simulink model "stellaris_test_buttons"  (R2012b)
settings: Solver=FixedStepDiscrete  SolverMode=SingleTasking  StartTime=0.0  StopTime=10.0  FixedStep=0.05  RelTol=1e-3
libraries: stellaris_lib x6, simulink x3
settings Model: Creator=peselnikmg  LastModifiedBy=peselnikmg
settings DataIOCC: SignalLoggingSaveFormat=ModelDataLogs
settings OptimizationCC: OptimizeModelRefInitCode=on  LifeSpan=1
settings HardwareCC: ProdEndianess=LittleEndian  ProdHWDeviceType=Texas Instruments->TMS470
settings RTWCC: SystemTargetFile=stellaris.tlc  TemplateMakefile=stellaris_tmf  PostCodeGenCommand=stellaris_customcode(buildInfo)  Description=TI Stellaris LaunchPad  GenerateReport=on  ProcessScript=stellaris_make_rtw_hook  IncludeHyperlinkInReport=on  GenerateTraceInfo=on  GenerateTraceReport=on  GenerateTraceReportSl=on  GenerateTraceReportSf=on  GenerateTraceReportEml=on  GenerateCodeMetricsReport=on  GenerateCodeReplacementReport=on
settings CodeAppCC: IgnoreCustomStorageClasses=off
settings STFCustomTargetCC: CodeReplacementLibrary=ANSI_C  CombineOutputUpdateFcns=on  ERTCustomFileBanners=on  SupportContinuousTime=off  SupportNonInlinedSFcns=off  GRTInterface=off  SystemTargetFile=stellaris.tlc
settings ERTTargetCC: CodeReplacementLibrary=ANSI_C  MultiwordLength=2048  ParMdlRefBuildCompliant=off  CompOptLevelCompliant=off  ConcurrentExecutionCompliant=off  ERTFirstTimeCompliant=off  ModelStepFunctionPrototypeControlCompliant=off  CPPClassGenCompliant=off  InlinedParameterPlacement=NonHierarchical  ERTCustomFileTemplate=stellaris_srmain.tlc  ConvertIfToSwitch=off  SuppressUnreachableDefaultCases=off

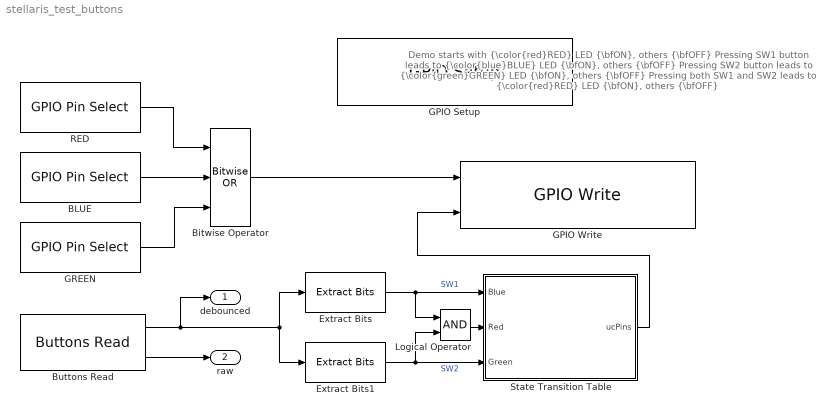
== system stellaris_test_buttons ==
  note: Demo starts with {\color{red}RED} LED {\bfON}, others {\bfOFF}
      |
      | Pressing SW1 button leads to {\color{blue}BLUE} LED {\bfON}, others {\bfOFF}
      | Pressing SW2 button leads to {\color{green}GREEN} LED {\bfON}, others {\bfOFF}
      | Pressing both SW1 and SW2 leads to {\color{red}RED} LED {\bfON}, others {\bfOFF}
  BLUE : stellaris_lib/GPIO/GPIO Pin Select  GPIO_PIN_X=GPIO_PIN_2
  Bitwise Operator : simulink/Logic and Bit Operations/Bitwise Operator  logicop=OR  UseBitMask=off  NumInputPorts=3  BitMask=bin2dec('11011001')  BitMaskRealWorld=Stored Integer
  Buttons Read : stellaris_lib/Buttons/Buttons Read
  Extract Bits : simulink/Logic and Bit Operations/Extract Bits  bitsToExtract=Range of bits  numBits=8  bitIdxRange=0  outScalingMode=Treat bit field as an integer
  Extract Bits1 : simulink/Logic and Bit Operations/Extract Bits  bitsToExtract=Range of bits  numBits=8  bitIdxRange=4  outScalingMode=Treat bit field as an integer
  GPIO Setup : stellaris_lib/GPIO/GPIO Setup  GPIO_PORTX_BASE=GPIO_PORTF_BASE  PinsOutput_0=Input  PinsOutput_1=Output  PinsOutput_2=Output  PinsOutput_3=Output  PinsOutput_4=Input  PinsOutput_5=Input  PinsOutput_6=Input  PinsOutput_7=Input
  GPIO Write : stellaris_lib/GPIO/GPIO Write  GPIO_PORTX_BASE=GPIO_PORTF_BASE
  GREEN : stellaris_lib/GPIO/GPIO Pin Select  GPIO_PIN_X=GPIO_PIN_3
  Logical Operator : Logic  AllPortsSameDT=off  OutDataTypeStr=boolean
  RED : stellaris_lib/GPIO/GPIO Pin Select  GPIO_PIN_X=GPIO_PIN_1
  State Transition Table : State Transition Table  TreatAsAtomicUnit=on
  debounced : Outport
  raw : Outport  Port=2
  wires:
  BLUE/1 -> Bitwise Operator/2
  RED/1 -> Bitwise Operator/1
  GREEN/1 -> Bitwise Operator/3
  Bitwise Operator/1 -> GPIO Write/1
  Buttons Read/1 -> Extract Bits1/1, Extract Bits/1, debounced/1
  Extract Bits1/1 -> Logical Operator/2, State Transition Table/3(Green)  "SW2"
  Extract Bits/1 -> Logical Operator/1, State Transition Table/1(Blue)  "SW1"
  Buttons Read/2 -> raw/1
  Logical Operator/1 -> State Transition Table/2(Red)
  State Transition Table/1(ucPins) -> GPIO Write/2

== stateflow chart stellaris_test_buttons/State Transition Table ==
  state RED
    du: ucPins = uint8(2);
  state GREEN
    du: ucPins = uint8(4);
  state BLUE
    du: ucPins = uint8(8);
  (default) -> RED
  (junction 30) -> RED
  RED -> (junction 24) [order 1] : [Blue > 0 && Green == 0]
  (junction 32) -> (junction 30)
  (junction 24) -> (junction 22)
  RED -> GREEN [order 2] : [Green > 0 && Blue == 0]
  GREEN -> RED [order 1] : [Red > 0]
  GREEN -> BLUE [order 2] : [Blue > 0]
  BLUE -> GREEN [order 2] : [Green > 0]
  BLUE -> (junction 32) [order 1] : [Red > 0]
  (junction 22) -> BLUE
  data: Blue input; Red input; Green input; ucPins output
